simulink model "AC_LADRC"  (R2023a)
settings: Solver=FixedStepDiscrete  StartTime=0.0  StopTime=10.0  FixedStep=1/400  RelTol=1e-3
undefined symbols (not defined in the file): AC_LADRC_b0, AC_LADRC_K_eso, AC_LADRC_W_c, ANG_PIT_P, ANG_RLL_P, ANG_YAW_P
libraries: slctrlblks x3
settings Model: Creator=30258  LastModifiedBy=30258
settings DataIOCC: ReturnWorkspaceOutputs=off
settings OptimizationCC: EnhancedBackFolding=on  PassReuseOutputArgsAs=Individual arguments  ZeroExternalMemoryAtStartup=off  ZeroInternalMemoryAtStartup=off  OptimizeBlockOrder=speed  DifferentSizesBufferReuse=on  OptimizationCustomize=off  EfficientTunableParamExpr=on
settings DebuggingCC: ParameterTunabilityLossMsg=error
settings HardwareCC: ProdBitPerPointer=32  ProdBitPerSizeT=32  ProdBitPerPtrDiffT=32  ProdLargestAtomicInteger=Long  ProdLargestAtomicFloat=Double  ProdWordSize=32  ProdHWDeviceType=ARM Compatible->ARM Cortex-M
settings SFSimCC: MATLABDynamicMemAlloc=off
settings RTWCC: Description=Embedded Coder  SystemTargetFile=ert.tlc  GenCodeOnly=on  PackageGeneratedCodeAndArtifacts=on  TemplateMakefile=ert_default_tmf  Toolchain=MinGW64 | gmake (64-bit Windows)  TargetLang=C++
settings CodeAppCC: ForceParamTrailComments=on  IgnoreCustomStorageClasses=off  OperatorAnnotations=on  SimulinkDataObjDesc=on  SFDataObjDesc=on  InsertBlockDesc=on
settings ERTTargetCC: TargetLangStandard=C++11 (ISO)  GenerateSampleERTMain=on  CodeInterfacePackaging=C++ class  SupportVariableSizeSignals=on  RootIOFormat=Structure reference  ERTCustomFileTemplate=example_file_process.tlc

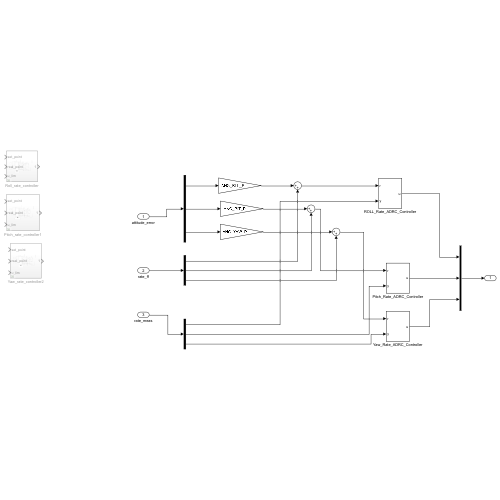
[thumbnail: Simulink's stored preview of the top-level diagram]
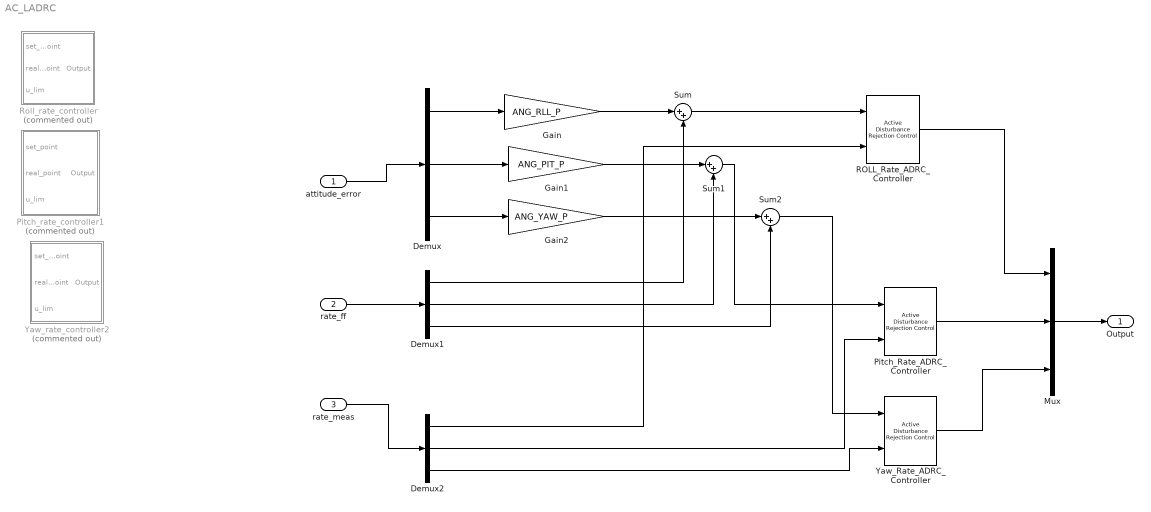
== system AC_LADRC ==
  attitude_error : Inport  OutDataTypeStr=single
  rate_ff : Inport  Port=2  OutDataTypeStr=single
  rate_meas : Inport  Port=3  OutDataTypeStr=single
  Demux : Demux  Outputs=3
  Demux1 : Demux  Outputs=3
  Demux2 : Demux  Outputs=3
  Gain : Gain  Gain=ANG_RLL_P  ParamDataTypeStr=single  OutDataTypeStr=single
  Gain1 : Gain  Gain=ANG_PIT_P  ParamDataTypeStr=single  OutDataTypeStr=single
  Gain2 : Gain  Gain=ANG_YAW_P  ParamDataTypeStr=single  OutDataTypeStr=single
  Mux : Mux  Inputs=3
  Pitch_Rate_ADRC_Controller : slctrlblks/Active Disturbance Rejection Control  time_domain=discrete-time  Ts=1/400  model_type=first-order  b0=PIT_B0  wc=PIT_Wc  wo=PIT_Wo  x0=0  ulim_checkbox=off  umax=inf  umin=-inf  xhat_checkbox=off
  Pitch_rate_controller1 : Subsystem  Commented=on
  ROLL_Rate_ADRC_Controller : slctrlblks/Active Disturbance Rejection Control  time_domain=discrete-time  Ts=1/400  model_type=first-order  b0=RLL_B0  wc=RLL_Wc  wo=RLL_Wo  x0=0  ulim_checkbox=off  umax=inf  umin=-inf  xhat_checkbox=off
  Roll_rate_controller : Subsystem  Commented=on
  Sum : Sum  Inputs=|++  AccumDataTypeStr=single  OutDataTypeStr=single
  Sum1 : Sum  Inputs=|++  AccumDataTypeStr=single  OutDataTypeStr=single
  Sum2 : Sum  Inputs=|++  AccumDataTypeStr=single  OutDataTypeStr=single
  Yaw_Rate_ADRC_Controller : slctrlblks/Active Disturbance Rejection Control  time_domain=discrete-time  Ts=1/400  model_type=first-order  b0=YAW_B0  wc=YAW_Wc  wo=YAW_Wo  x0=0  ulim_checkbox=off  umax=inf  umin=-inf  xhat_checkbox=off
  Yaw_rate_controller2 : Subsystem  Commented=on
  Output : Outport  OutDataTypeStr=single
  wires:
  attitude_error/1 -> Demux/1
  rate_ff/1 -> Demux1/1
  rate_meas/1 -> Demux2/1
  ROLL_Rate_ADRC_Controller/1 -> Mux/1
  Pitch_Rate_ADRC_Controller/1 -> Mux/2
  Yaw_Rate_ADRC_Controller/1 -> Mux/3
  Demux/1 -> Gain/1
  Demux1/1 -> Sum/2
  Gain/1 -> Sum/1
  Demux2/1 -> ROLL_Rate_ADRC_Controller/2
  Sum/1 -> ROLL_Rate_ADRC_Controller/1
  Demux/2 -> Gain1/1
  Demux/3 -> Gain2/1
  Gain1/1 -> Sum1/1
  Demux1/2 -> Sum1/2
  Sum1/1 -> Pitch_Rate_ADRC_Controller/1
  Demux2/2 -> Pitch_Rate_ADRC_Controller/2
  Gain2/1 -> Sum2/1
  Demux2/3 -> Yaw_Rate_ADRC_Controller/2
  Sum2/1 -> Yaw_Rate_ADRC_Controller/1
  Demux1/3 -> Sum2/2
  Mux/1 -> Output/1

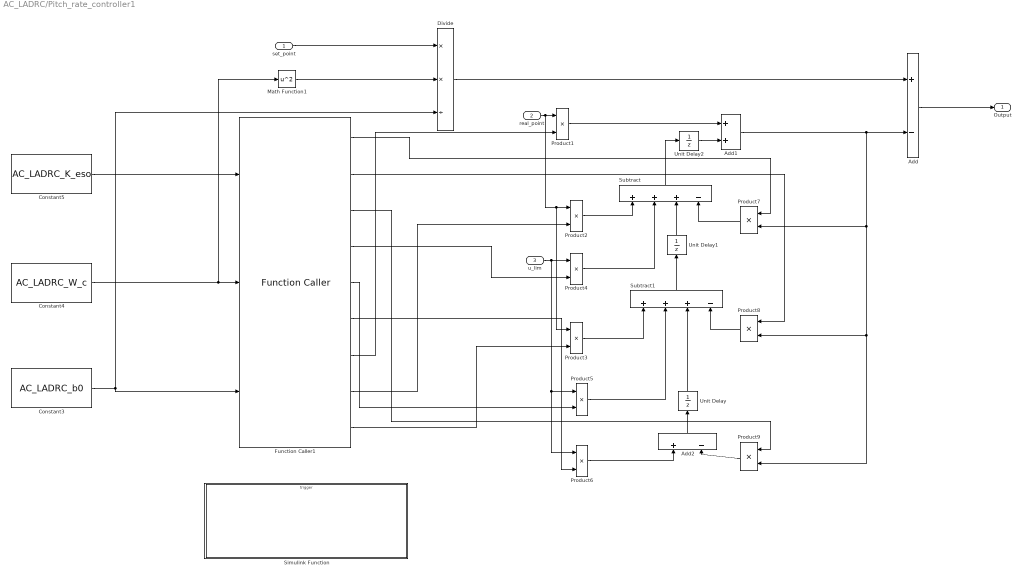
== system AC_LADRC/Pitch_rate_controller1 ==
  set_point : Inport  OutDataTypeStr=single
  real_point : Inport  Port=2  OutDataTypeStr=single
  u_lim : Inport  Port=3  OutDataTypeStr=single
  Add : Sum  Inputs=+-  AccumDataTypeStr=single  OutDataTypeStr=single
  Add1 : Sum
  Add2 : Sum  Inputs=+-  AccumDataTypeStr=single  OutDataTypeStr=single
  Constant3 : Constant  Value=AC_LADRC_b0  OutDataTypeStr=single  SampleTime=1/400
  Constant4 : Constant  Value=AC_LADRC_W_c  OutDataTypeStr=single  SampleTime=1/400
  Constant5 : Constant  Value=AC_LADRC_K_eso  OutDataTypeStr=single  SampleTime=1/400
  Divide : Product  Inputs=**/  OutDataTypeStr=single
  Function Caller1 : FunctionCaller  FunctionPrototype=[y,y1,y2,y3,y4,y5,y6,y7,y8] = f_Ladrc_para(u,u1,u2)  InputArgumentSpecifications=<Enter example>  OutputArgumentSpecifications=<Enter example>
  Math Function1 : Math  Operator=square  SignedPower=on  OutputSignalType=real  OutDataTypeStr=single  RndMeth=Zero
  Product{1..2,4,7} (4 alike) : Product
  Product{3,5..6,8..9} (5 alike) : Product  OutDataTypeStr=single
  Simulink Function : Subsystem  TreatAsAtomicUnit=on
  Subtract : Sum  Inputs=+++-  OutDataTypeStr=single
  Subtract1 : Sum  Inputs=+++-  OutDataTypeStr=single
  Unit Delay : UnitDelay  SampleTime=1/400  HasFrameUpgradeWarning=on
  Unit Delay1 : UnitDelay  SampleTime=1/400  HasFrameUpgradeWarning=on
  Unit Delay2 : UnitDelay  SampleTime=1/400  HasFrameUpgradeWarning=on
  Output : Outport  OutDataTypeStr=single
  wires:
  Constant4/1 -> Function Caller1/2, Math Function1/1
  Add1/1 -> Product9/2, Product8/2, Product7/2, Add/2
  Unit Delay2/1 -> Add1/2
  u_lim/1 -> Product6/1, Product5/1, Product4/1
  real_point/1 -> Product3/1, Product2/1, Product1/1
  Function Caller1/1 -> Product7/1
  Product7/1 -> Subtract/4
  Constant3/1 -> Function Caller1/3, Divide/3
  Constant5/1 -> Function Caller1/1
  Function Caller1/7 -> Product1/2
  Product8/1 -> Subtract1/4
  Function Caller1/4 -> Product4/2
  Function Caller1/8 -> Product2/2
  Product6/1 -> Add2/1
  Function Caller1/5 -> Product5/2
  Divide/1 -> Add/1
  Product3/1 -> Subtract1/1
  set_point/1 -> Divide/1
  Product4/1 -> Subtract/2
  Product5/1 -> Subtract1/2
  Add/1 -> Output/1
  Unit Delay/1 -> Subtract1/3
  Function Caller1/6 -> Product6/2
  Product1/1 -> Add1/1
  Function Caller1/9 -> Product3/2
  Product9/1 -> Add2/2
  Add2/1 -> Unit Delay/1
  Function Caller1/3 -> Product9/1
  Function Caller1/2 -> Product8/1
  Math Function1/1 -> Divide/2
  Unit Delay1/1 -> Subtract/3
  Product2/1 -> Subtract/1
  Subtract1/1 -> Unit Delay1/1
  Subtract/1 -> Unit Delay2/1

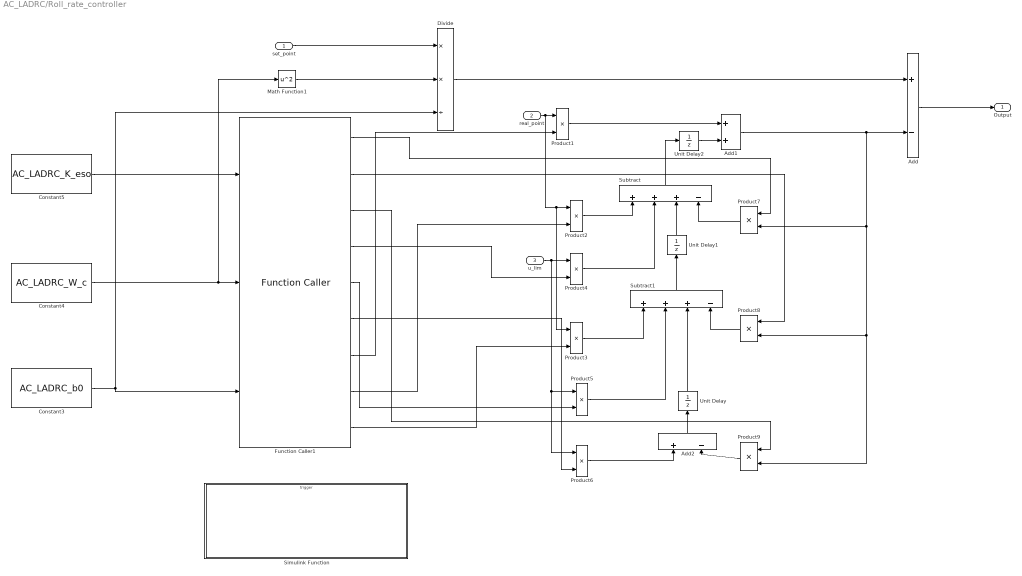
== system AC_LADRC/Roll_rate_controller ==
  set_point : Inport  OutDataTypeStr=single
  real_point : Inport  Port=2  OutDataTypeStr=single
  u_lim : Inport  Port=3  OutDataTypeStr=single
  Add : Sum  Inputs=+-  AccumDataTypeStr=single  OutDataTypeStr=single
  Add1 : Sum
  Add2 : Sum  Inputs=+-  AccumDataTypeStr=single  OutDataTypeStr=single
  Constant3 : Constant  Value=AC_LADRC_b0  OutDataTypeStr=single  SampleTime=1/400
  Constant4 : Constant  Value=AC_LADRC_W_c  OutDataTypeStr=single  SampleTime=1/400
  Constant5 : Constant  Value=AC_LADRC_K_eso  OutDataTypeStr=single  SampleTime=1/400
  Divide : Product  Inputs=**/  OutDataTypeStr=single
  Function Caller1 : FunctionCaller  FunctionPrototype=[y,y1,y2,y3,y4,y5,y6,y7,y8] = f_Ladrc_para(u,u1,u2)  InputArgumentSpecifications=<Enter example>  OutputArgumentSpecifications=<Enter example>
  Math Function1 : Math  Operator=square  SignedPower=on  OutputSignalType=real  OutDataTypeStr=single  RndMeth=Zero
  Product{1..2,4,7} (4 alike) : Product
  Product{3,5..6,8..9} (5 alike) : Product  OutDataTypeStr=single
  Simulink Function : Subsystem  TreatAsAtomicUnit=on
  Subtract : Sum  Inputs=+++-  OutDataTypeStr=single
  Subtract1 : Sum  Inputs=+++-  OutDataTypeStr=single
  Unit Delay : UnitDelay  SampleTime=1/400  HasFrameUpgradeWarning=on
  Unit Delay1 : UnitDelay  SampleTime=1/400  HasFrameUpgradeWarning=on
  Unit Delay2 : UnitDelay  SampleTime=1/400  HasFrameUpgradeWarning=on
  Output : Outport  OutDataTypeStr=single
  wires:
  Constant4/1 -> Function Caller1/2, Math Function1/1
  Add1/1 -> Product9/2, Product8/2, Product7/2, Add/2
  Unit Delay2/1 -> Add1/2
  u_lim/1 -> Product6/1, Product5/1, Product4/1
  real_point/1 -> Product3/1, Product2/1, Product1/1
  Function Caller1/1 -> Product7/1
  Product7/1 -> Subtract/4
  Constant3/1 -> Function Caller1/3, Divide/3
  Constant5/1 -> Function Caller1/1
  Function Caller1/7 -> Product1/2
  Product8/1 -> Subtract1/4
  Function Caller1/4 -> Product4/2
  Function Caller1/8 -> Product2/2
  Product6/1 -> Add2/1
  Function Caller1/5 -> Product5/2
  Divide/1 -> Add/1
  Product3/1 -> Subtract1/1
  set_point/1 -> Divide/1
  Product4/1 -> Subtract/2
  Product5/1 -> Subtract1/2
  Add/1 -> Output/1
  Unit Delay/1 -> Subtract1/3
  Function Caller1/6 -> Product6/2
  Product1/1 -> Add1/1
  Function Caller1/9 -> Product3/2
  Product9/1 -> Add2/2
  Add2/1 -> Unit Delay/1
  Function Caller1/3 -> Product9/1
  Function Caller1/2 -> Product8/1
  Math Function1/1 -> Divide/2
  Unit Delay1/1 -> Subtract/3
  Product2/1 -> Subtract/1
  Subtract1/1 -> Unit Delay1/1
  Subtract/1 -> Unit Delay2/1

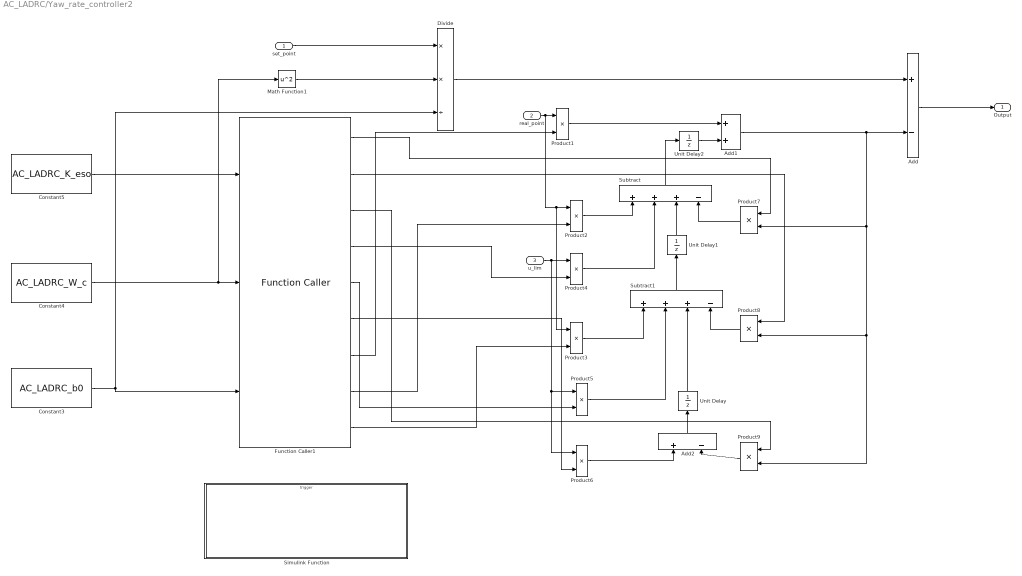
== system AC_LADRC/Yaw_rate_controller2 ==
  set_point : Inport  OutDataTypeStr=single
  real_point : Inport  Port=2  OutDataTypeStr=single
  u_lim : Inport  Port=3  OutDataTypeStr=single
  Add : Sum  Inputs=+-  AccumDataTypeStr=single  OutDataTypeStr=single
  Add1 : Sum
  Add2 : Sum  Inputs=+-  AccumDataTypeStr=single  OutDataTypeStr=single
  Constant3 : Constant  Value=AC_LADRC_b0  OutDataTypeStr=single  SampleTime=1/400
  Constant4 : Constant  Value=AC_LADRC_W_c  OutDataTypeStr=single  SampleTime=1/400
  Constant5 : Constant  Value=AC_LADRC_K_eso  OutDataTypeStr=single  SampleTime=1/400
  Divide : Product  Inputs=**/  OutDataTypeStr=single
  Function Caller1 : FunctionCaller  FunctionPrototype=[y,y1,y2,y3,y4,y5,y6,y7,y8] = f_Ladrc_para(u,u1,u2)  InputArgumentSpecifications=<Enter example>  OutputArgumentSpecifications=<Enter example>
  Math Function1 : Math  Operator=square  SignedPower=on  OutputSignalType=real  OutDataTypeStr=single  RndMeth=Zero
  Product{1..2,4,7} (4 alike) : Product
  Product{3,5..6,8..9} (5 alike) : Product  OutDataTypeStr=single
  Simulink Function : Subsystem  TreatAsAtomicUnit=on
  Subtract : Sum  Inputs=+++-  OutDataTypeStr=single
  Subtract1 : Sum  Inputs=+++-  OutDataTypeStr=single
  Unit Delay : UnitDelay  SampleTime=1/400  HasFrameUpgradeWarning=on
  Unit Delay1 : UnitDelay  SampleTime=1/400  HasFrameUpgradeWarning=on
  Unit Delay2 : UnitDelay  SampleTime=1/400  HasFrameUpgradeWarning=on
  Output : Outport  OutDataTypeStr=single
  wires:
  Constant4/1 -> Function Caller1/2, Math Function1/1
  Add1/1 -> Product9/2, Product8/2, Product7/2, Add/2
  Unit Delay2/1 -> Add1/2
  u_lim/1 -> Product6/1, Product5/1, Product4/1
  real_point/1 -> Product3/1, Product2/1, Product1/1
  Function Caller1/1 -> Product7/1
  Product7/1 -> Subtract/4
  Constant3/1 -> Function Caller1/3, Divide/3
  Constant5/1 -> Function Caller1/1
  Function Caller1/7 -> Product1/2
  Product8/1 -> Subtract1/4
  Function Caller1/4 -> Product4/2
  Function Caller1/8 -> Product2/2
  Product6/1 -> Add2/1
  Function Caller1/5 -> Product5/2
  Divide/1 -> Add/1
  Product3/1 -> Subtract1/1
  set_point/1 -> Divide/1
  Product4/1 -> Subtract/2
  Product5/1 -> Subtract1/2
  Add/1 -> Output/1
  Unit Delay/1 -> Subtract1/3
  Function Caller1/6 -> Product6/2
  Product1/1 -> Add1/1
  Function Caller1/9 -> Product3/2
  Product9/1 -> Add2/2
  Add2/1 -> Unit Delay/1
  Function Caller1/3 -> Product9/1
  Function Caller1/2 -> Product8/1
  Math Function1/1 -> Divide/2
  Unit Delay1/1 -> Subtract/3
  Product2/1 -> Subtract/1
  Subtract1/1 -> Unit Delay1/1
  Subtract/1 -> Unit Delay2/1

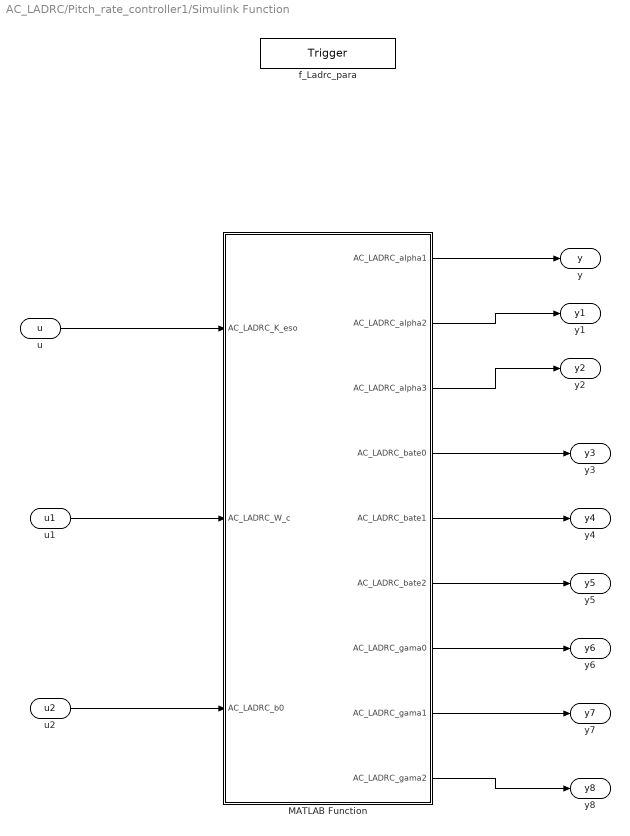
== system AC_LADRC/Pitch_rate_controller1/Simulink Function ==
  f_Ladrc_para : TriggerPort  TriggerType=function-call  IsSimulinkFunction=on  FunctionName=f_Ladrc_para  FunctionVisibility=scoped  VariantControl=(inherit)
  MATLAB Function : MATLAB Function  TreatAsAtomicUnit=on
  u : ArgIn  DisableCoverage=on  OutDataTypeStr=single  ArgumentName=u
  u1 : ArgIn  DisableCoverage=on  Port=2  OutDataTypeStr=single  ArgumentName=u1
  u2 : ArgIn  DisableCoverage=on  Port=3  OutDataTypeStr=single  ArgumentName=u2
  y : ArgOut  DisableCoverage=on  OutDataTypeStr=single  ArgumentName=y
  y1 : ArgOut  DisableCoverage=on  Port=2  OutDataTypeStr=single  ArgumentName=y1
  y2 : ArgOut  DisableCoverage=on  Port=3  OutDataTypeStr=single  ArgumentName=y2
  y3 : ArgOut  DisableCoverage=on  Port=4  OutDataTypeStr=single  ArgumentName=y3
  y4 : ArgOut  DisableCoverage=on  Port=5  OutDataTypeStr=single  ArgumentName=y4
  y5 : ArgOut  DisableCoverage=on  Port=6  OutDataTypeStr=single  ArgumentName=y5
  y6 : ArgOut  DisableCoverage=on  Port=7  OutDataTypeStr=single  ArgumentName=y6
  y7 : ArgOut  DisableCoverage=on  Port=8  OutDataTypeStr=single  ArgumentName=y7
  y8 : ArgOut  DisableCoverage=on  Port=9  OutDataTypeStr=single  ArgumentName=y8
  wires:
  u/1 -> MATLAB Function/1(AC_LADRC_K_eso)
  MATLAB Function/1(AC_LADRC_alpha1) -> y/1
  u2/1 -> MATLAB Function/3(AC_LADRC_b0)
  u1/1 -> MATLAB Function/2(AC_LADRC_W_c)
  MATLAB Function/2(AC_LADRC_alpha2) -> y1/1
  MATLAB Function/3(AC_LADRC_alpha3) -> y2/1
  MATLAB Function/4(AC_LADRC_bate0) -> y3/1
  MATLAB Function/5(AC_LADRC_bate1) -> y4/1
  MATLAB Function/6(AC_LADRC_bate2) -> y5/1
  MATLAB Function/7(AC_LADRC_gama0) -> y6/1
  MATLAB Function/8(AC_LADRC_gama1) -> y7/1
  MATLAB Function/9(AC_LADRC_gama2) -> y8/1

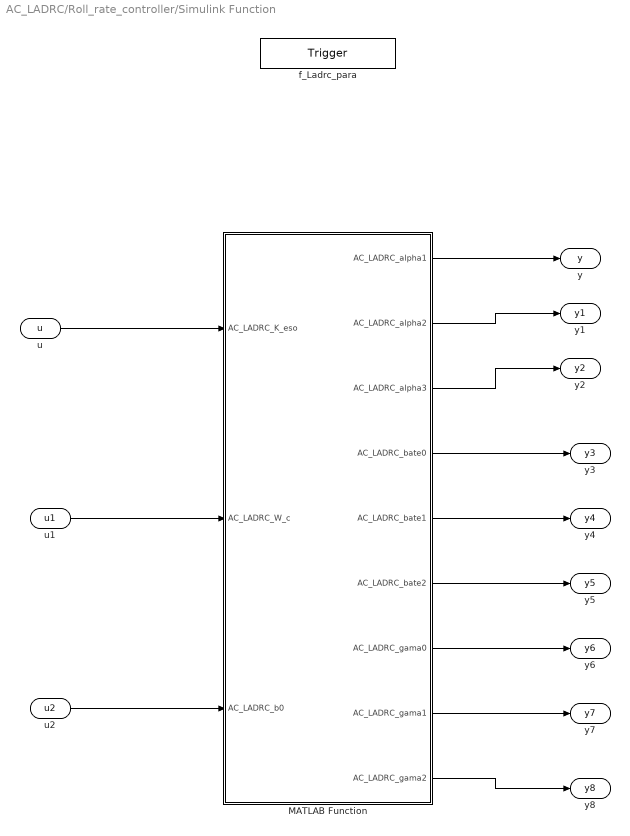
== system AC_LADRC/Roll_rate_controller/Simulink Function ==
  f_Ladrc_para : TriggerPort  TriggerType=function-call  IsSimulinkFunction=on  FunctionName=f_Ladrc_para  FunctionVisibility=scoped  VariantControl=(inherit)
  MATLAB Function : MATLAB Function  TreatAsAtomicUnit=on
  u : ArgIn  DisableCoverage=on  OutDataTypeStr=single  ArgumentName=u
  u1 : ArgIn  DisableCoverage=on  Port=2  OutDataTypeStr=single  ArgumentName=u1
  u2 : ArgIn  DisableCoverage=on  Port=3  OutDataTypeStr=single  ArgumentName=u2
  y : ArgOut  DisableCoverage=on  OutDataTypeStr=single  ArgumentName=y
  y1 : ArgOut  DisableCoverage=on  Port=2  OutDataTypeStr=single  ArgumentName=y1
  y2 : ArgOut  DisableCoverage=on  Port=3  OutDataTypeStr=single  ArgumentName=y2
  y3 : ArgOut  DisableCoverage=on  Port=4  OutDataTypeStr=single  ArgumentName=y3
  y4 : ArgOut  DisableCoverage=on  Port=5  OutDataTypeStr=single  ArgumentName=y4
  y5 : ArgOut  DisableCoverage=on  Port=6  OutDataTypeStr=single  ArgumentName=y5
  y6 : ArgOut  DisableCoverage=on  Port=7  OutDataTypeStr=single  ArgumentName=y6
  y7 : ArgOut  DisableCoverage=on  Port=8  OutDataTypeStr=single  ArgumentName=y7
  y8 : ArgOut  DisableCoverage=on  Port=9  OutDataTypeStr=single  ArgumentName=y8
  wires:
  u/1 -> MATLAB Function/1(AC_LADRC_K_eso)
  MATLAB Function/1(AC_LADRC_alpha1) -> y/1
  u2/1 -> MATLAB Function/3(AC_LADRC_b0)
  u1/1 -> MATLAB Function/2(AC_LADRC_W_c)
  MATLAB Function/2(AC_LADRC_alpha2) -> y1/1
  MATLAB Function/3(AC_LADRC_alpha3) -> y2/1
  MATLAB Function/4(AC_LADRC_bate0) -> y3/1
  MATLAB Function/5(AC_LADRC_bate1) -> y4/1
  MATLAB Function/6(AC_LADRC_bate2) -> y5/1
  MATLAB Function/7(AC_LADRC_gama0) -> y6/1
  MATLAB Function/8(AC_LADRC_gama1) -> y7/1
  MATLAB Function/9(AC_LADRC_gama2) -> y8/1

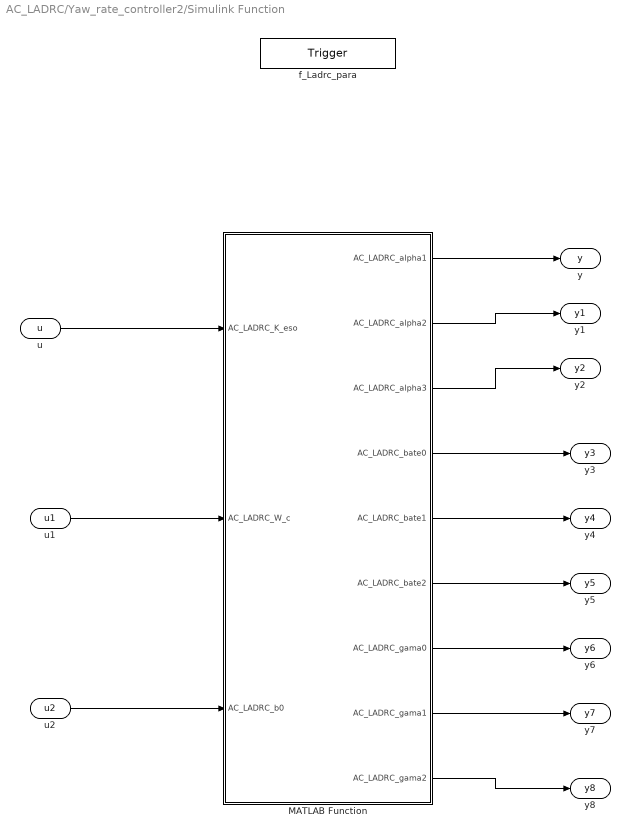
== system AC_LADRC/Yaw_rate_controller2/Simulink Function ==
  f_Ladrc_para : TriggerPort  TriggerType=function-call  IsSimulinkFunction=on  FunctionName=f_Ladrc_para  FunctionVisibility=scoped  VariantControl=(inherit)
  MATLAB Function : MATLAB Function  TreatAsAtomicUnit=on
  u : ArgIn  DisableCoverage=on  OutDataTypeStr=single  ArgumentName=u
  u1 : ArgIn  DisableCoverage=on  Port=2  OutDataTypeStr=single  ArgumentName=u1
  u2 : ArgIn  DisableCoverage=on  Port=3  OutDataTypeStr=single  ArgumentName=u2
  y : ArgOut  DisableCoverage=on  OutDataTypeStr=single  ArgumentName=y
  y1 : ArgOut  DisableCoverage=on  Port=2  OutDataTypeStr=single  ArgumentName=y1
  y2 : ArgOut  DisableCoverage=on  Port=3  OutDataTypeStr=single  ArgumentName=y2
  y3 : ArgOut  DisableCoverage=on  Port=4  OutDataTypeStr=single  ArgumentName=y3
  y4 : ArgOut  DisableCoverage=on  Port=5  OutDataTypeStr=single  ArgumentName=y4
  y5 : ArgOut  DisableCoverage=on  Port=6  OutDataTypeStr=single  ArgumentName=y5
  y6 : ArgOut  DisableCoverage=on  Port=7  OutDataTypeStr=single  ArgumentName=y6
  y7 : ArgOut  DisableCoverage=on  Port=8  OutDataTypeStr=single  ArgumentName=y7
  y8 : ArgOut  DisableCoverage=on  Port=9  OutDataTypeStr=single  ArgumentName=y8
  wires:
  u/1 -> MATLAB Function/1(AC_LADRC_K_eso)
  MATLAB Function/1(AC_LADRC_alpha1) -> y/1
  u2/1 -> MATLAB Function/3(AC_LADRC_b0)
  u1/1 -> MATLAB Function/2(AC_LADRC_W_c)
  MATLAB Function/2(AC_LADRC_alpha2) -> y1/1
  MATLAB Function/3(AC_LADRC_alpha3) -> y2/1
  MATLAB Function/4(AC_LADRC_bate0) -> y3/1
  MATLAB Function/5(AC_LADRC_bate1) -> y4/1
  MATLAB Function/6(AC_LADRC_bate2) -> y5/1
  MATLAB Function/7(AC_LADRC_gama0) -> y6/1
  MATLAB Function/8(AC_LADRC_gama1) -> y7/1
  MATLAB Function/9(AC_LADRC_gama2) -> y8/1

== matlab function AC_LADRC/Roll_rate_controller/Simulink Function/MATLAB Function ==
  data: AC_LADRC_K_eso input; AC_LADRC_alpha1 output; AC_LADRC_W_c input; AC_LADRC_b0 input; AC_LADRC_alpha2 output; AC_LADRC_alpha3 output; AC_LADRC_bate0 output; AC_LADRC_bate1 output; AC_LADRC_bate2 output; AC_LADRC_gama0 output; AC_LADRC_gama1 output; AC_LADRC_gama2 output
function [AC_LADRC_alpha1,AC_LADRC_alpha2,AC_LADRC_alpha3,AC_LADRC_bate0,AC_LADRC_bate1,AC_LADRC_bate2,AC_LADRC_gama0,AC_LADRC_gama1,AC_LADRC_gama2] = fcn(AC_LADRC_K_eso,AC_LADRC_W_c,AC_LADRC_b0)
AP_LADRC_T=1/400;
AP_LADRC_Z_eso=eps^(-AC_LADRC_K_eso*AC_LADRC_W_c*AP_LADRC_T);
AC_LADRC_alpha1=-3*AP_LADRC_Z_eso;
AC_LADRC_alpha2=3*AP_LADRC_Z_eso^2;
AC_LADRC_alpha3=-AP_LADRC_Z_eso^3;
AC_LADRC_bate0=(-AP_LADRC_T*AC_LADRC_W_c*AP_LADRC_Z_eso^3*(4-AP_LADRC_T*AC_LADRC_W_c)+AP_LADRC_T*AC_LADRC_W_c*(1+AP_LADRC_Z_eso)^3-(1-AP_LADRC_Z_eso)^3)/2;
AC_LADRC_bate1=(-AP_LADRC_T*AC_LADRC_W_c*(1+AP_LADRC_Z_eso)^3-(1-AP_LADRC_Z_eso)^3)/2;
AC_LADRC_bate2=(AP_LADRC_T*AC_LADRC_W_c*AP_LADRC_Z_eso^3*(4-AP_LADRC_T*AC_LADRC_W_c))/2;
AC_LADRC_gama0=(AP_LADRC_T^2*AC_LADRC_W_c^2*(1-AP_LADRC_Z_eso^3)+3*AP_LADRC_T*AC_LADRC_W_c*(1-AP_LADRC_Z_eso-AP_LADRC_Z_eso^2+AP_LADRC_Z_eso^3)+(1-AP_LADRC_Z_eso)^3)/(AC_LADRC_b0*AP_LADRC_T^2);
AC_LADRC_gama1=(3*AP_LADRC_T^2*AC_LADRC_W_c^2*(-AP_LADRC_Z_eso+AP_LADRC_Z_eso^3)+4*AP_LADRC_T*AC_LADRC_W_c*(-1+3*AP_LADRC_Z_eso^2-2*AP_LADRC_Z_eso^3)-2*(1-AP_LADRC_Z_eso)^3)/(AC_LADRC_b0*AP_LADRC_T^2);
AC_LADRC_gama2=(3*AP_LADRC_T^2*AC_LADRC_W_c^2*(AP_LADRC_Z_eso^2+AP_LADRC_Z_eso^3)+AP_LADRC_T*AC_LADRC_W_c*(1+3*AP_LADRC_Z_eso+9*AP_LADRC_Z_eso^2+5*AP_LADRC_Z_eso^3)+(1-AP_LADRC_Z_eso)^3)/(AC_LADRC_b0*AP_LADRC_T^2);

== matlab function AC_LADRC/Pitch_rate_controller1/Simulink Function/MATLAB Function ==
  data: AC_LADRC_K_eso input; AC_LADRC_alpha1 output; AC_LADRC_W_c input; AC_LADRC_b0 input; AC_LADRC_alpha2 output; AC_LADRC_alpha3 output; AC_LADRC_bate0 output; AC_LADRC_bate1 output; AC_LADRC_bate2 output; AC_LADRC_gama0 output; AC_LADRC_gama1 output; AC_LADRC_gama2 output
function [AC_LADRC_alpha1,AC_LADRC_alpha2,AC_LADRC_alpha3,AC_LADRC_bate0,AC_LADRC_bate1,AC_LADRC_bate2,AC_LADRC_gama0,AC_LADRC_gama1,AC_LADRC_gama2] = fcn(AC_LADRC_K_eso,AC_LADRC_W_c,AC_LADRC_b0)
AP_LADRC_T=1/400;
AP_LADRC_Z_eso=eps^(-AC_LADRC_K_eso*AC_LADRC_W_c*AP_LADRC_T);
AC_LADRC_alpha1=-3*AP_LADRC_Z_eso;
AC_LADRC_alpha2=3*AP_LADRC_Z_eso^2;
AC_LADRC_alpha3=-AP_LADRC_Z_eso^3;
AC_LADRC_bate0=(-AP_LADRC_T*AC_LADRC_W_c*AP_LADRC_Z_eso^3*(4-AP_LADRC_T*AC_LADRC_W_c)+AP_LADRC_T*AC_LADRC_W_c*(1+AP_LADRC_Z_eso)^3-(1-AP_LADRC_Z_eso)^3)/2;
AC_LADRC_bate1=(-AP_LADRC_T*AC_LADRC_W_c*(1+AP_LADRC_Z_eso)^3-(1-AP_LADRC_Z_eso)^3)/2;
AC_LADRC_bate2=(AP_LADRC_T*AC_LADRC_W_c*AP_LADRC_Z_eso^3*(4-AP_LADRC_T*AC_LADRC_W_c))/2;
AC_LADRC_gama0=(AP_LADRC_T^2*AC_LADRC_W_c^2*(1-AP_LADRC_Z_eso^3)+3*AP_LADRC_T*AC_LADRC_W_c*(1-AP_LADRC_Z_eso-AP_LADRC_Z_eso^2+AP_LADRC_Z_eso^3)+(1-AP_LADRC_Z_eso)^3)/(AC_LADRC_b0*AP_LADRC_T^2);
AC_LADRC_gama1=(3*AP_LADRC_T^2*AC_LADRC_W_c^2*(-AP_LADRC_Z_eso+AP_LADRC_Z_eso^3)+4*AP_LADRC_T*AC_LADRC_W_c*(-1+3*AP_LADRC_Z_eso^2-2*AP_LADRC_Z_eso^3)-2*(1-AP_LADRC_Z_eso)^3)/(AC_LADRC_b0*AP_LADRC_T^2);
AC_LADRC_gama2=(3*AP_LADRC_T^2*AC_LADRC_W_c^2*(AP_LADRC_Z_eso^2+AP_LADRC_Z_eso^3)+AP_LADRC_T*AC_LADRC_W_c*(1+3*AP_LADRC_Z_eso+9*AP_LADRC_Z_eso^2+5*AP_LADRC_Z_eso^3)+(1-AP_LADRC_Z_eso)^3)/(AC_LADRC_b0*AP_LADRC_T^2);

== matlab function AC_LADRC/Yaw_rate_controller2/Simulink Function/MATLAB Function ==
  data: AC_LADRC_K_eso input; AC_LADRC_alpha1 output; AC_LADRC_W_c input; AC_LADRC_b0 input; AC_LADRC_alpha2 output; AC_LADRC_alpha3 output; AC_LADRC_bate0 output; AC_LADRC_bate1 output; AC_LADRC_bate2 output; AC_LADRC_gama0 output; AC_LADRC_gama1 output; AC_LADRC_gama2 output
function [AC_LADRC_alpha1,AC_LADRC_alpha2,AC_LADRC_alpha3,AC_LADRC_bate0,AC_LADRC_bate1,AC_LADRC_bate2,AC_LADRC_gama0,AC_LADRC_gama1,AC_LADRC_gama2] = fcn(AC_LADRC_K_eso,AC_LADRC_W_c,AC_LADRC_b0)
AP_LADRC_T=1/400;
AP_LADRC_Z_eso=eps^(-AC_LADRC_K_eso*AC_LADRC_W_c*AP_LADRC_T);
AC_LADRC_alpha1=-3*AP_LADRC_Z_eso;
AC_LADRC_alpha2=3*AP_LADRC_Z_eso^2;
AC_LADRC_alpha3=-AP_LADRC_Z_eso^3;
AC_LADRC_bate0=(-AP_LADRC_T*AC_LADRC_W_c*AP_LADRC_Z_eso^3*(4-AP_LADRC_T*AC_LADRC_W_c)+AP_LADRC_T*AC_LADRC_W_c*(1+AP_LADRC_Z_eso)^3-(1-AP_LADRC_Z_eso)^3)/2;
AC_LADRC_bate1=(-AP_LADRC_T*AC_LADRC_W_c*(1+AP_LADRC_Z_eso)^3-(1-AP_LADRC_Z_eso)^3)/2;
AC_LADRC_bate2=(AP_LADRC_T*AC_LADRC_W_c*AP_LADRC_Z_eso^3*(4-AP_LADRC_T*AC_LADRC_W_c))/2;
AC_LADRC_gama0=(AP_LADRC_T^2*AC_LADRC_W_c^2*(1-AP_LADRC_Z_eso^3)+3*AP_LADRC_T*AC_LADRC_W_c*(1-AP_LADRC_Z_eso-AP_LADRC_Z_eso^2+AP_LADRC_Z_eso^3)+(1-AP_LADRC_Z_eso)^3)/(AC_LADRC_b0*AP_LADRC_T^2);
AC_LADRC_gama1=(3*AP_LADRC_T^2*AC_LADRC_W_c^2*(-AP_LADRC_Z_eso+AP_LADRC_Z_eso^3)+4*AP_LADRC_T*AC_LADRC_W_c*(-1+3*AP_LADRC_Z_eso^2-2*AP_LADRC_Z_eso^3)-2*(1-AP_LADRC_Z_eso)^3)/(AC_LADRC_b0*AP_LADRC_T^2);
AC_LADRC_gama2=(3*AP_LADRC_T^2*AC_LADRC_W_c^2*(AP_LADRC_Z_eso^2+AP_LADRC_Z_eso^3)+AP_LADRC_T*AC_LADRC_W_c*(1+3*AP_LADRC_Z_eso+9*AP_LADRC_Z_eso^2+5*AP_LADRC_Z_eso^3)+(1-AP_LADRC_Z_eso)^3)/(AC_LADRC_b0*AP_LADRC_T^2);
